simulink model "untuned_filter"  (R2021a)
settings: Solver=VariableStepAuto  StartTime=0.0  StopTime=10.0  RelTol=1e-3
libraries: xbsIndex_r4 x753
(part 1 of 2)
settings Model: Creator=s4671313  LastModifiedBy=s4671313

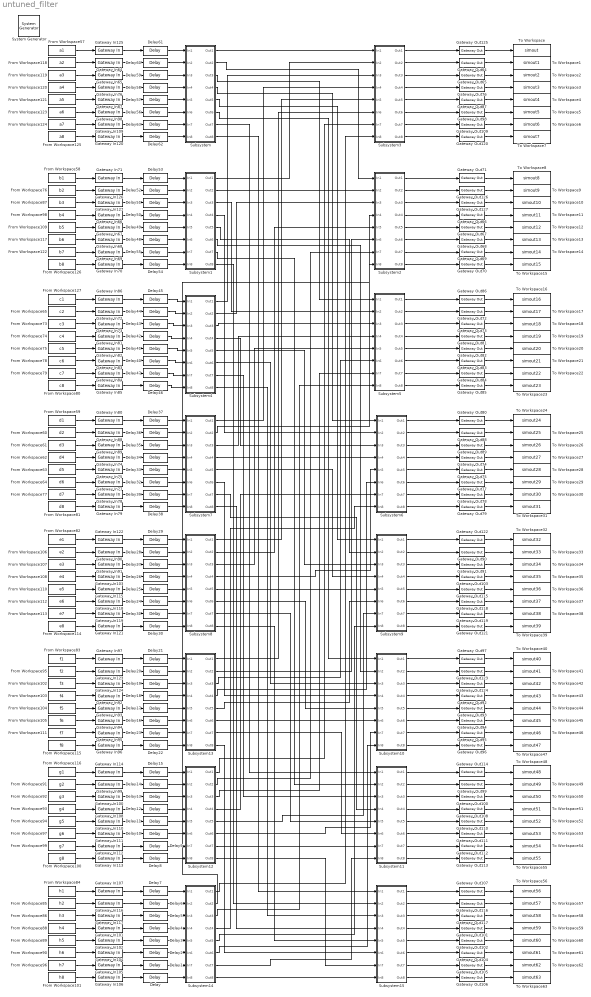
== system untuned_filter ==
  " System Generator" : xbsIndex_r4/ System Generator  Tag=genX  xilinxfamily=artix7  part=xc7a200t  speed=-2  package=fbg676  synthesis_tool=Vivado  clock_wrapper=Clock Enables  directory=./netlist  proj_type=Vivado  Synth_file=Vivado Synthesis Defaults  Impl_file=Vivado Implementation Defaults  testbench=off  simulink_period=1  sysclk_period=10  dcm_input_clock_period=10  incr_netlist=off  trim_vbits=Everywhere in SubSystem  dbl_ovrd=According to Block Masks  core_generation=According to Block Masks  run_coregen=off  deprecated_control=off  eval_field=0  block_type=sysgen
  Delay{,1..63} (64 alike) : xbsIndex_r4/Delay  rst=off  infoeditControl=Selection of Reset will increase slice count due to use of real FFs and instead of SRLs  en=off  latency=1  reg_retiming=off  dbl_ovrd=off  block_type=delay
  From Workspace100 : FromWorkspace  VariableName=g8
  From Workspace101 : FromWorkspace  VariableName=h8
  From Workspace102 : FromWorkspace  VariableName=f3
  From Workspace103 : FromWorkspace  VariableName=f4
  From Workspace104 : FromWorkspace  VariableName=f5
  From Workspace105 : FromWorkspace  VariableName=f6
  From Workspace106 : FromWorkspace  VariableName=e2
  From Workspace107 : FromWorkspace  VariableName=e3
  From Workspace108 : FromWorkspace  VariableName=e4
  From Workspace109 : FromWorkspace  VariableName=b5
  From Workspace110 : FromWorkspace  VariableName=e5
  From Workspace111 : FromWorkspace  VariableName=f7
  From Workspace112 : FromWorkspace  VariableName=e6
  From Workspace113 : FromWorkspace  VariableName=e7
  From Workspace114 : FromWorkspace  VariableName=e8
  From Workspace115 : FromWorkspace  VariableName=f8
  From Workspace116 : FromWorkspace  VariableName=g1
  From Workspace117 : FromWorkspace  VariableName=b6
  From Workspace118 : FromWorkspace  VariableName=a2
  From Workspace119 : FromWorkspace  VariableName=a3
  From Workspace120 : FromWorkspace  VariableName=a4
  From Workspace121 : FromWorkspace  VariableName=a5
  From Workspace122 : FromWorkspace  VariableName=b7
  From Workspace123 : FromWorkspace  VariableName=a6
  From Workspace124 : FromWorkspace  VariableName=a7
  From Workspace125 : FromWorkspace  VariableName=a8
  From Workspace126 : FromWorkspace  VariableName=b8
  From Workspace127 : FromWorkspace  VariableName=c1
  From Workspace57 : FromWorkspace  VariableName=a1
  From Workspace58 : FromWorkspace  VariableName=b1
  From Workspace59 : FromWorkspace  VariableName=d1
  From Workspace60 : FromWorkspace  VariableName=d2
  From Workspace61 : FromWorkspace  VariableName=d3
  From Workspace62 : FromWorkspace  VariableName=d4
  From Workspace63 : FromWorkspace  VariableName=d5
  From Workspace64 : FromWorkspace  VariableName=d6
  From Workspace65 : FromWorkspace  VariableName=c2
  From Workspace73 : FromWorkspace  VariableName=c3
  From Workspace74 : FromWorkspace  VariableName=c4
  From Workspace75 : FromWorkspace  VariableName=c5
  From Workspace76 : FromWorkspace  VariableName=b2
  From Workspace77 : FromWorkspace  VariableName=d7
  From Workspace78 : FromWorkspace  VariableName=c6
  From Workspace79 : FromWorkspace  VariableName=c7
  From Workspace80 : FromWorkspace  VariableName=c8
  From Workspace81 : FromWorkspace  VariableName=d8
  From Workspace82 : FromWorkspace  VariableName=e1
  From Workspace83 : FromWorkspace  VariableName=f1
  From Workspace84 : FromWorkspace  VariableName=h1
  From Workspace85 : FromWorkspace  VariableName=h2
  From Workspace86 : FromWorkspace  VariableName=h3
  From Workspace87 : FromWorkspace  VariableName=b3
  From Workspace88 : FromWorkspace  VariableName=h4
  From Workspace89 : FromWorkspace  VariableName=h5
  From Workspace90 : FromWorkspace  VariableName=h6
  From Workspace91 : FromWorkspace  VariableName=g2
  From Workspace92 : FromWorkspace  VariableName=g3
  From Workspace93 : FromWorkspace  VariableName=g4
  From Workspace94 : FromWorkspace  VariableName=g5
  From Workspace95 : FromWorkspace  VariableName=f2
  From Workspace96 : FromWorkspace  VariableName=h7
  From Workspace97 : FromWorkspace  VariableName=g6
  From Workspace98 : FromWorkspace  VariableName=b4
  From Workspace99 : FromWorkspace  VariableName=g7
  Gateway In{64..127} (64 alike) : xbsIndex_r4/Gateway In  gui_display_data_type=Fixed-point  arith_type="Signed  (2's comp)"  n_bits=W  bin_pt=D  preci_type=Single  exp_width=8  frac_width=24  rows=1  columns=1  quantization="Round  (unbiased: +/- Inf)"  overflow=Saturate  period=1  UseAsADC=off  ADCChannel='1'  interface=None  automatic_assignment=on  address_offset=hex2dec('00')  intf_name=''  intf_description=''  default_value=0  timing_constraint=None  locs_specified=off  LOCs={}  io_standard={}  inherit_from_input=off  hdl_port=on  dbl_ovrd=off  block_type=gatewayin
  Gateway Out{64..127} (64 alike) : xbsIndex_r4/Gateway Out  inherit_from_input=off  hdl_port=on  rows=1  columns=1  UseAsDAC=off  DACChannel='1'  interface=None  automatic_assignment=on  address_offset=hex2dec('00')  intf_name=''  intf_description=''  timing_constraint=None  locs_specified=off  LOCs={}  io_standard={}  block_type=gatewayout
  Subsystem : Subsystem
  Subsystem1 : Subsystem
  Subsystem10 : Subsystem
  Subsystem11 : Subsystem
  Subsystem12 : Subsystem
  Subsystem13 : Subsystem
  Subsystem14 : Subsystem
  Subsystem15 : Subsystem
  Subsystem2 : Subsystem
  Subsystem3 : Subsystem
  Subsystem4 : Subsystem
  Subsystem5 : Subsystem
  Subsystem6 : Subsystem
  Subsystem7 : Subsystem
  Subsystem8 : Subsystem
  Subsystem9 : Subsystem
  To Workspace : ToWorkspace  VariableName=simout  SampleTime=-1
  To Workspace1 : ToWorkspace  VariableName=simout1  SampleTime=-1
  To Workspace10 : ToWorkspace  VariableName=simout10  SampleTime=-1
  To Workspace11 : ToWorkspace  VariableName=simout11  SampleTime=-1
  To Workspace12 : ToWorkspace  VariableName=simout12  SampleTime=-1
  To Workspace13 : ToWorkspace  VariableName=simout13  SampleTime=-1
  To Workspace14 : ToWorkspace  VariableName=simout14  SampleTime=-1
  To Workspace15 : ToWorkspace  VariableName=simout15  SampleTime=-1
  To Workspace16 : ToWorkspace  VariableName=simout16  SampleTime=-1
  To Workspace17 : ToWorkspace  VariableName=simout17  SampleTime=-1
  To Workspace18 : ToWorkspace  VariableName=simout18  SampleTime=-1
  To Workspace19 : ToWorkspace  VariableName=simout19  SampleTime=-1
  To Workspace2 : ToWorkspace  VariableName=simout2  SampleTime=-1
  To Workspace20 : ToWorkspace  VariableName=simout20  SampleTime=-1
  To Workspace21 : ToWorkspace  VariableName=simout21  SampleTime=-1
  To Workspace22 : ToWorkspace  VariableName=simout22  SampleTime=-1
  To Workspace23 : ToWorkspace  VariableName=simout23  SampleTime=-1
  To Workspace24 : ToWorkspace  VariableName=simout24  SampleTime=-1
  To Workspace25 : ToWorkspace  VariableName=simout25  SampleTime=-1
  To Workspace26 : ToWorkspace  VariableName=simout26  SampleTime=-1
  To Workspace27 : ToWorkspace  VariableName=simout27  SampleTime=-1
  To Workspace28 : ToWorkspace  VariableName=simout28  SampleTime=-1
  To Workspace29 : ToWorkspace  VariableName=simout29  SampleTime=-1
  To Workspace3 : ToWorkspace  VariableName=simout3  SampleTime=-1
  To Workspace30 : ToWorkspace  VariableName=simout30  SampleTime=-1
  To Workspace31 : ToWorkspace  VariableName=simout31  SampleTime=-1
  To Workspace32 : ToWorkspace  VariableName=simout32  SampleTime=-1
  To Workspace33 : ToWorkspace  VariableName=simout33  SampleTime=-1
  To Workspace34 : ToWorkspace  VariableName=simout34  SampleTime=-1
  To Workspace35 : ToWorkspace  VariableName=simout35  SampleTime=-1
  To Workspace36 : ToWorkspace  VariableName=simout36  SampleTime=-1
  To Workspace37 : ToWorkspace  VariableName=simout37  SampleTime=-1
  To Workspace38 : ToWorkspace  VariableName=simout38  SampleTime=-1
  To Workspace39 : ToWorkspace  VariableName=simout39  SampleTime=-1
  To Workspace4 : ToWorkspace  VariableName=simout4  SampleTime=-1
  To Workspace40 : ToWorkspace  VariableName=simout40  SampleTime=-1
  To Workspace41 : ToWorkspace  VariableName=simout41  SampleTime=-1
  To Workspace42 : ToWorkspace  VariableName=simout42  SampleTime=-1
  To Workspace43 : ToWorkspace  VariableName=simout43  SampleTime=-1
  To Workspace44 : ToWorkspace  VariableName=simout44  SampleTime=-1
  To Workspace45 : ToWorkspace  VariableName=simout45  SampleTime=-1
  To Workspace46 : ToWorkspace  VariableName=simout46  SampleTime=-1
  To Workspace47 : ToWorkspace  VariableName=simout47  SampleTime=-1
  To Workspace48 : ToWorkspace  VariableName=simout48  SampleTime=-1
  To Workspace49 : ToWorkspace  VariableName=simout49  SampleTime=-1
  To Workspace5 : ToWorkspace  VariableName=simout5  SampleTime=-1
  To Workspace50 : ToWorkspace  VariableName=simout50  SampleTime=-1
  To Workspace51 : ToWorkspace  VariableName=simout51  SampleTime=-1
  To Workspace52 : ToWorkspace  VariableName=simout52  SampleTime=-1
  To Workspace53 : ToWorkspace  VariableName=simout53  SampleTime=-1
  To Workspace54 : ToWorkspace  VariableName=simout54  SampleTime=-1
  To Workspace55 : ToWorkspace  VariableName=simout55  SampleTime=-1
  To Workspace56 : ToWorkspace  VariableName=simout56  SampleTime=-1
  To Workspace57 : ToWorkspace  VariableName=simout57  SampleTime=-1
  To Workspace58 : ToWorkspace  VariableName=simout58  SampleTime=-1
  To Workspace59 : ToWorkspace  VariableName=simout59  SampleTime=-1
  To Workspace6 : ToWorkspace  VariableName=simout6  SampleTime=-1
  To Workspace60 : ToWorkspace  VariableName=simout60  SampleTime=-1
  To Workspace61 : ToWorkspace  VariableName=simout61  SampleTime=-1
  To Workspace62 : ToWorkspace  VariableName=simout62  SampleTime=-1
  To Workspace63 : ToWorkspace  VariableName=simout63  SampleTime=-1
  To Workspace7 : ToWorkspace  VariableName=simout7  SampleTime=-1
  To Workspace8 : ToWorkspace  VariableName=simout8  SampleTime=-1
  To Workspace9 : ToWorkspace  VariableName=simout9  SampleTime=-1
  wires:
  Subsystem15/5(Out5) -> Gateway Out102/1
  Subsystem15/4(Out4) -> Gateway Out101/1
  Subsystem15/3(Out3) -> Gateway Out117/1
  Subsystem15/2(Out2) -> Gateway Out116/1
  Subsystem1/8(Out8) -> Subsystem15/2(In2)
  Subsystem12/8(Out8) -> Subsystem15/7(In7)
  Subsystem8/8(Out8) -> Subsystem15/5(In5)
  Subsystem/8(Out8) -> Subsystem15/1(In1)
  Subsystem15/8(Out8) -> Gateway Out106/1
  Subsystem4/2(Out2) -> Subsystem2/3(In3)
  Delay3/1 -> Subsystem14/5(In5)
  Delay/1 -> Subsystem14/8(In8)
  Delay6/1 -> Subsystem14/2(In2)
  Subsystem14/1(Out1) -> Subsystem3/8(In8)
  Subsystem4/3(Out3) -> Subsystem5/3(In3)
  Subsystem1/7(Out7) -> Subsystem11/2(In2)
  Subsystem7/8(Out8) -> Subsystem15/4(In4)
  Subsystem13/7(Out7) -> Subsystem11/6(In6)
  Subsystem/7(Out7) -> Subsystem11/1(In1)
  Delay46/1 -> Subsystem4/8(In8)
  Subsystem4/6(Out6) -> Subsystem10/3(In3)
  Subsystem4/4(Out4) -> Subsystem6/3(In3)
  Subsystem14/3(Out3) -> Subsystem5/8(In8)
  Delay40/1 -> Subsystem4/6(In6)
  Delay43/1 -> Subsystem4/3(In3)
  Delay9/1 -> Subsystem12/7(In7)
  Delay12/1 -> Subsystem12/4(In4)
  Delay10/1 -> Subsystem12/6(In6)
  Delay14/1 -> Subsystem12/2(In2)
  Delay11/1 -> Subsystem12/5(In5)
  Subsystem12/5(Out5) -> Subsystem9/7(In7)
  Subsystem12/1(Out1) -> Subsystem3/7(In7)
  Delay41/1 -> Subsystem4/5(In5)
  Delay2/1 -> Subsystem14/6(In6)
  Subsystem14/6(Out6) -> Subsystem10/8(In8)
  Subsystem12/6(Out6) -> Subsystem10/7(In7)
  Subsystem14/4(Out4) -> Subsystem6/8(In8)
  Subsystem12/2(Out2) -> Subsystem2/7(In7)
  Subsystem8/6(Out6) -> Subsystem10/5(In5)
  Subsystem/6(Out6) -> Subsystem10/1(In1)
  Subsystem1/6(Out6) -> Subsystem10/2(In2)
  Subsystem10/8(Out8) -> Gateway Out96/1
  Subsystem10/4(Out4) -> Gateway Out92/1
  Subsystem10/2(Out2) -> Gateway Out123/1
  Subsystem10/3(Out3) -> Gateway Out124/1
  Subsystem13/6(Out6) -> Subsystem10/6(In6)
  Subsystem13/3(Out3) -> Subsystem5/6(In6)
  Subsystem13/1(Out1) -> Subsystem3/6(In6)
  Delay17/1 -> Subsystem13/5(In5)
  Delay16/1 -> Subsystem13/6(In6)
  Delay22/1 -> Subsystem13/8(In8)
  Subsystem10/1(Out1) -> Gateway Out97/1
  Delay27/1 -> Subsystem8/3(In3)
  Delay28/1 -> Subsystem8/2(In2)
  Subsystem8/1(Out1) -> Subsystem3/5(In5)
  Subsystem7/7(Out7) -> Subsystem11/4(In4)
  Delay24/1 -> Subsystem8/6(In6)
  Subsystem6/2(Out2) -> Gateway Out88/1
  Subsystem15/6(Out6) -> Gateway Out104/1
  Subsystem6/7(Out7) -> Gateway Out78/1
  Subsystem6/8(Out8) -> Gateway Out79/1
  Subsystem6/3(Out3) -> Gateway Out89/1
  Subsystem6/6(Out6) -> Gateway Out77/1
  Subsystem6/1(Out1) -> Gateway Out80/1
  Subsystem1/4(Out4) -> Subsystem6/2(In2)
  Subsystem7/4(Out4) -> Subsystem6/4(In4)
  Delay29/1 -> Subsystem8/1(In1)
  Subsystem13/5(Out5) -> Subsystem9/6(In6)
  Delay21/1 -> Subsystem13/1(In1)
  Subsystem13/4(Out4) -> Subsystem6/6(In6)
  Delay18/1 -> Subsystem13/4(In4)
  Subsystem1/1(Out1) -> Subsystem3/2(In2)
  Delay54/1 -> Subsystem1/8(In8)
  Subsystem1/2(Out2) -> Subsystem2/2(In2)
  Delay51/1 -> Subsystem1/3(In3)
  Delay55/1 -> Subsystem1/7(In7)
  Delay52/1 -> Subsystem1/2(In2)
  Subsystem5/5(Out5) -> Gateway Out82/1
  Subsystem8/4(Out4) -> Subsystem6/5(In5)
  Subsystem5/4(Out4) -> Gateway Out81/1
  Subsystem5/2(Out2) -> Gateway Out72/1
  Subsystem5/3(Out3) -> Gateway Out73/1
  Delay1/1 -> Subsystem14/7(In7)
  Delay39/1 -> Subsystem7/7(In7)
  Gateway In64/1 -> Delay60/1
  Subsystem8/2(Out2) -> Subsystem2/5(In5)
  Gateway In109/1 -> Delay63/1
  Gateway In87/1 -> Delay57/1
  Gateway In83/1 -> Delay40/1
  Gateway In85/1 -> Delay46/1
  Gateway In84/1 -> Delay47/1
  Subsystem3/3(Out3) -> Gateway Out65/1
  Gateway In72/1 -> Delay44/1
  Gateway In82/1 -> Delay41/1
  Gateway In86/1 -> Delay45/1
  Subsystem3/8(Out8) -> Gateway Out120/1
  Gateway In67/1 -> Delay49/1
  Gateway In113/1 -> Delay8/1
  Gateway In100/1 -> Delay13/1
  Gateway In114/1 -> Delay15/1
  Subsystem2/4(Out4) -> Gateway Out66/1
  Subsystem2/1(Out1) -> Gateway Out71/1
  Gateway In108/1 -> Delay12/1
  Subsystem2/8(Out8) -> Gateway Out70/1
  Gateway In112/1 -> Delay9/1
  Gateway In110/1 -> Delay11/1
  Delay44/1 -> Subsystem4/2(In2)
  Delay7/1 -> Subsystem14/1(In1)
  Gateway In99/1 -> Delay14/1
  Delay8/1 -> Subsystem12/8(In8)
  Gateway In104/1 -> Delay2/1
  Gateway In81/1 -> Delay42/1
  Gateway In102/1 -> Delay3/1
  Subsystem9/6(Out6) -> Gateway Out118/1
  Subsystem9/5(Out5) -> Gateway Out115/1
  Gateway In115/1 -> Delay25/1
  Gateway In90/1 -> Delay28/1
  Gateway In122/1 -> Delay29/1
  Gateway In116/1 -> Delay6/1
  Gateway In107/1 -> Delay7/1
  Subsystem3/6(Out6) -> Gateway Out98/1
  Gateway In88/1 -> Delay36/1
  Gateway In89/1 -> Delay35/1
  Gateway In77/1 -> Delay32/1
  Gateway In80/1 -> Delay37/1
  Gateway In78/1 -> Delay39/1
  Gateway In124/1 -> Delay19/1
  Gateway In95/1 -> Delay23/1
  Gateway In96/1 -> Delay22/1
  Gateway In127/1 -> Delay51/1
  Gateway In68/1 -> Delay48/1
  Subsystem2/5(Out5) -> Gateway Out67/1
  Subsystem/3(Out3) -> Subsystem5/1(In1)
  Subsystem/2(Out2) -> Subsystem2/1(In1)
  Subsystem6/4(Out4) -> Gateway Out74/1
  Subsystem2/6(Out6) -> Gateway Out68/1
  Delay23/1 -> Subsystem13/7(In7)
  Gateway In93/1 -> Delay17/1
  Delay63/1 -> Subsystem/7(In7)
  Delay56/1 -> Subsystem/6(In6)
  Delay57/1 -> Subsystem/5(In5)
  Subsystem13/8(Out8) -> Subsystem15/6(In6)
  Delay60/1 -> Subsystem/2(In2)
  Gateway In74/1 -> Delay34/1
  Gateway In106/1 -> Delay/1
  Subsystem7/1(Out1) -> Subsystem3/4(In4)
  Delay61/1 -> Subsystem/1(In1)
  Delay37/1 -> Subsystem7/1(In1)
  Subsystem14/8(Out8) -> Subsystem15/8(In8)
  Delay34/1 -> Subsystem7/4(In4)
  Delay31/1 -> Subsystem8/7(In7)
  Delay36/1 -> Subsystem7/2(In2)
  Subsystem5/1(Out1) -> Gateway Out86/1
  Delay62/1 -> Subsystem/8(In8)
  Subsystem3/5(Out5) -> Gateway Out87/1
  Subsystem/1(Out1) -> Subsystem3/1(In1)
  Gateway In76/1 -> Delay58/1
  Subsystem3/4(Out4) -> Gateway Out76/1
  Subsystem3/2(Out2) -> Gateway Out64/1
  Gateway In94/1 -> Delay16/1
  Subsystem15/1(Out1) -> Gateway Out107/1
  Delay45/1 -> Subsystem4/1(In1)
  Delay47/1 -> Subsystem4/7(In7)
  Gateway In125/1 -> Delay61/1
  Subsystem11/2(Out2) -> Gateway Out99/1
  Subsystem9/2(Out2) -> Gateway Out90/1
  Subsystem11/3(Out3) -> Gateway Out100/1
  Subsystem11/5(Out5) -> Gateway Out110/1
  Gateway In123/1 -> Delay20/1
  Gateway In65/1 -> Delay59/1
  Subsystem11/8(Out8) -> Gateway Out113/1
  Subsystem9/4(Out4) -> Gateway Out103/1
  Gateway In120/1 -> Delay62/1
  Subsystem11/4(Out4) -> Gateway Out108/1
  Gateway In101/1 -> Delay4/1
  Delay58/1 -> Subsystem/4(In4)
  Subsystem5/6(Out6) -> Gateway Out83/1
  Subsystem12/7(Out7) -> Subsystem11/7(In7)
  Subsystem5/8(Out8) -> Gateway Out85/1
  Delay50/1 -> Subsystem1/4(In4)
  Subsystem5/7(Out7) -> Gateway Out84/1
  Gateway In70/1 -> Delay54/1
  Delay49/1 -> Subsystem1/5(In5)
  Subsystem1/3(Out3) -> Subsystem5/2(In2)
  Delay20/1 -> Subsystem13/2(In2)
  Gateway In121/1 -> Delay30/1
  Subsystem13/2(Out2) -> Subsystem2/6(In6)
  Subsystem8/3(Out3) -> Subsystem5/5(In5)
  Subsystem14/7(Out7) -> Subsystem11/8(In8)
  Subsystem3/7(Out7) -> Gateway Out109/1
  Gateway In103/1 -> Delay26/1
  Subsystem2/3(Out3) -> Gateway Out127/1
  Subsystem9/1(Out1) -> Gateway Out122/1
  Subsystem/4(Out4) -> Subsystem6/1(In1)
  Subsystem7/5(Out5) -> Subsystem9/4(In4)
  Subsystem11/6(Out6) -> Gateway Out111/1
  Delay42/1 -> Subsystem4/4(In4)
  Gateway Out102/1 -> To Workspace60/1
  Gateway In75/1 -> Delay33/1
  Gateway Out103/1 -> To Workspace35/1
  Subsystem10/5(Out5) -> Gateway Out93/1
  From Workspace65/1 -> Gateway In72/1
  Subsystem4/7(Out7) -> Subsystem11/3(In3)
  Gateway Out104/1 -> To Workspace61/1
  Gateway In111/1 -> Delay10/1
  Gateway Out107/1 -> To Workspace56/1
  Gateway Out124/1 -> To Workspace42/1
  Gateway In98/1 -> Delay56/1
  Gateway Out64/1 -> To Workspace1/1
  Subsystem8/5(Out5) -> Subsystem9/5(In5)
  Gateway Out66/1 -> To Workspace11/1
  From Workspace121/1 -> Gateway In87/1
  From Workspace116/1 -> Gateway In114/1
  From Workspace96/1 -> Gateway In105/1
  Gateway Out96/1 -> To Workspace47/1
  From Workspace113/1 -> Gateway In119/1
  From Workspace61/1 -> Gateway In89/1
  From Workspace76/1 -> Gateway In126/1
  Gateway Out117/1 -> To Workspace58/1
  Gateway In117/1 -> Delay5/1
  Gateway Out84/1 -> To Workspace22/1
  Delay53/1 -> Subsystem1/1(In1)
  Subsystem12/3(Out3) -> Subsystem5/7(In7)
  From Workspace127/1 -> Gateway In86/1
  Gateway Out77/1 -> To Workspace29/1
  From Workspace115/1 -> Gateway In96/1
  Gateway Out116/1 -> To Workspace57/1
  From Workspace120/1 -> Gateway In76/1
  Delay15/1 -> Subsystem12/1(In1)
  From Workspace89/1 -> Gateway In102/1
  Gateway In118/1 -> Delay24/1
  Subsystem12/4(Out4) -> Subsystem6/7(In7)
  Gateway Out95/1 -> To Workspace46/1
  Gateway Out120/1 -> To Workspace7/1
  From Workspace114/1 -> Gateway In121/1
  From Workspace83/1 -> Gateway In97/1
  From Workspace62/1 -> Gateway In74/1
  Delay32/1 -> Subsystem7/6(In6)
  Gateway In79/1 -> Delay38/1
  From Workspace119/1 -> Gateway In65/1
  Gateway Out85/1 -> To Workspace23/1
  From Workspace59/1 -> Gateway In80/1
  From Workspace63/1 -> Gateway In75/1
  Gateway Out81/1 -> To Workspace19/1
  Subsystem2/7(Out7) -> Gateway Out69/1
  Subsystem15/7(Out7) -> Gateway Out105/1
  From Workspace88/1 -> Gateway In101/1
  From Workspace111/1 -> Gateway In95/1
  Gateway Out90/1 -> To Workspace33/1
  Subsystem4/1(Out1) -> Subsystem3/3(In3)
  From Workspace95/1 -> Gateway In123/1
  Subsystem4/8(Out8) -> Subsystem15/3(In3)
  From Workspace58/1 -> Gateway In71/1
  Gateway Out106/1 -> To Workspace63/1
  Subsystem8/7(Out7) -> Subsystem11/5(In5)
  From Workspace92/1 -> Gateway In100/1
  From Workspace101/1 -> Gateway In106/1
  Gateway Out99/1 -> To Workspace49/1
  Gateway Out78/1 -> To Workspace30/1
  Gateway Out83/1 -> To Workspace21/1
  From Workspace94/1 -> Gateway In110/1
  Gateway In105/1 -> Delay1/1
  From Workspace123/1 -> Gateway In98/1
  From Workspace91/1 -> Gateway In99/1
  Gateway Out93/1 -> To Workspace44/1
  From Workspace77/1 -> Gateway In78/1
  Gateway In97/1 -> Delay21/1
  From Workspace74/1 -> Gateway In81/1
  Subsystem10/7(Out7) -> Gateway Out95/1
  Gateway Out115/1 -> To Workspace36/1
  Delay26/1 -> Subsystem8/4(In4)
  Gateway Out91/1 -> To Workspace34/1
  From Workspace122/1 -> Gateway In69/1
  Gateway Out118/1 -> To Workspace37/1
  From Workspace79/1 -> Gateway In84/1
  Subsystem7/6(Out6) -> Subsystem10/4(In4)
  Gateway Out114/1 -> To Workspace48/1
  From Workspace112/1 -> Gateway In118/1
  From Workspace106/1 -> Gateway In90/1
  Gateway In119/1 -> Delay31/1
  Gateway Out108/1 -> To Workspace51/1
  Gateway Out119/1 -> To Workspace38/1
  Gateway Out105/1 -> To Workspace62/1
  Gateway Out65/1 -> To Workspace2/1
  Gateway Out101/1 -> To Workspace59/1
  Delay35/1 -> Subsystem7/3(In3)
  From Workspace107/1 -> Gateway In91/1
  From Workspace80/1 -> Gateway In85/1
  Gateway Out100/1 -> To Workspace50/1
  Gateway Out82/1 -> To Workspace20/1
  Subsystem14/5(Out5) -> Subsystem9/8(In8)
  Subsystem4/5(Out5) -> Subsystem9/3(In3)
  Gateway Out73/1 -> To Workspace18/1
  Delay5/1 -> Subsystem14/3(In3)
  From Workspace73/1 -> Gateway In73/1
  Gateway Out72/1 -> To Workspace17/1
  Gateway In73/1 -> Delay43/1
  From Workspace109/1 -> Gateway In67/1
  Subsystem6/5(Out5) -> Gateway Out75/1
  From Workspace104/1 -> Gateway In93/1
  Gateway Out92/1 -> To Workspace43/1
  From Workspace84/1 -> Gateway In107/1
  Subsystem1/5(Out5) -> Subsystem9/2(In2)
  Delay59/1 -> Subsystem/3(In3)
  Gateway Out70/1 -> To Workspace15/1
  Gateway In69/1 -> Delay55/1
  Gateway Out121/1 -> To Workspace39/1
  Subsystem/5(Out5) -> Subsystem9/1(In1)
  From Workspace105/1 -> Gateway In94/1
  From Workspace108/1 -> Gateway In103/1
  Gateway Out86/1 -> To Workspace16/1
  From Workspace110/1 -> Gateway In115/1
  Gateway Out71/1 -> To Workspace8/1
  From Workspace86/1 -> Gateway In117/1
  Subsystem9/7(Out7) -> Gateway Out119/1
  Gateway Out75/1 -> To Workspace28/1
  Gateway Out79/1 -> To Workspace31/1
  From Workspace99/1 -> Gateway In112/1
  Subsystem3/1(Out1) -> Gateway Out125/1
  Delay30/1 -> Subsystem8/8(In8)
  Gateway Out88/1 -> To Workspace25/1
  From Workspace125/1 -> Gateway In120/1
  Gateway Out122/1 -> To Workspace32/1
  Gateway In71/1 -> Delay53/1
  Subsystem7/3(Out3) -> Subsystem5/4(In4)
  Subsystem9/3(Out3) -> Gateway Out91/1
  From Workspace118/1 -> Gateway In64/1
  Gateway Out110/1 -> To Workspace52/1
  Subsystem2/2(Out2) -> Gateway Out126/1
  From Workspace100/1 -> Gateway In113/1
  Gateway Out94/1 -> To Workspace45/1
  Gateway Out67/1 -> To Workspace12/1
  Gateway Out98/1 -> To Workspace5/1
  From Workspace102/1 -> Gateway In124/1
  Gateway Out125/1 -> To Workspace/1
  Subsystem11/7(Out7) -> Gateway Out112/1
  From Workspace64/1 -> Gateway In77/1
  From Workspace87/1 -> Gateway In127/1
  Delay4/1 -> Subsystem14/4(In4)
  Gateway Out97/1 -> To Workspace40/1
  Subsystem7/2(Out2) -> Subsystem2/4(In4)
  From Workspace126/1 -> Gateway In70/1
  Subsystem10/6(Out6) -> Gateway Out94/1
  Gateway Out126/1 -> To Workspace9/1
  Subsystem11/1(Out1) -> Gateway Out114/1
  Delay33/1 -> Subsystem7/5(In5)
  From Workspace98/1 -> Gateway In66/1
  From Workspace124/1 -> Gateway In109/1
  Delay25/1 -> Subsystem8/5(In5)
  From Workspace103/1 -> Gateway In92/1
  From Workspace90/1 -> Gateway In104/1
  Subsystem14/2(Out2) -> Subsystem2/8(In8)
  Gateway Out113/1 -> To Workspace55/1
  Gateway In91/1 -> Delay27/1
  Gateway Out112/1 -> To Workspace54/1
  Gateway Out68/1 -> To Workspace13/1
  Delay13/1 -> Subsystem12/3(In3)
  Gateway Out76/1 -> To Workspace3/1
  From Workspace97/1 -> Gateway In111/1
  From Workspace93/1 -> Gateway In108/1
  From Workspace81/1 -> Gateway In79/1
  From Workspace85/1 -> Gateway In116/1
  From Workspace82/1 -> Gateway In122/1
  Gateway Out123/1 -> To Workspace41/1
  Delay38/1 -> Subsystem7/8(In8)
  Gateway Out87/1 -> To Workspace4/1
  Gateway Out111/1 -> To Workspace53/1
  Gateway In66/1 -> Delay50/1
  Subsystem9/8(Out8) -> Gateway Out121/1
  Delay48/1 -> Subsystem1/6(In6)
  Gateway Out109/1 -> To Workspace6/1
  Gateway In92/1 -> Delay18/1
  From Workspace57/1 -> Gateway In125/1
  Gateway Out74/1 -> To Workspace27/1
  Gateway Out89/1 -> To Workspace26/1
  From Workspace75/1 -> Gateway In82/1
  Gateway Out127/1 -> To Workspace10/1
  From Workspace78/1 -> Gateway In83/1
  From Workspace60/1 -> Gateway In88/1
  Delay19/1 -> Subsystem13/3(In3)
  Gateway Out80/1 -> To Workspace24/1
  Gateway Out69/1 -> To Workspace14/1
  Gateway In126/1 -> Delay52/1
  From Workspace117/1 -> Gateway In68/1

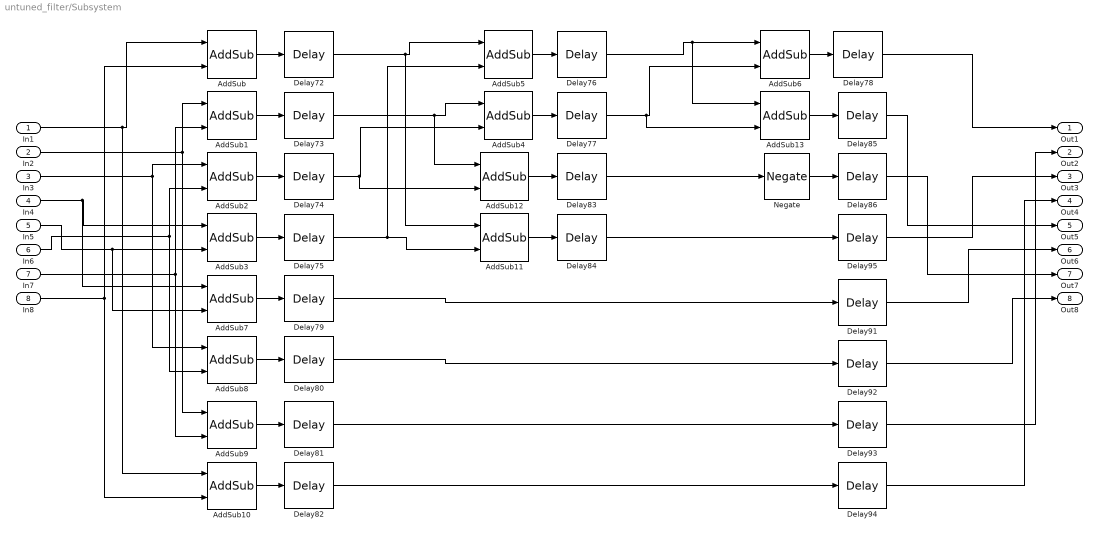
== system untuned_filter/Subsystem ==
  In1 : Inport
  In2 : Inport  Port=2
  In3 : Inport  Port=3
  In4 : Inport  Port=4
  In5 : Inport  Port=5
  In6 : Inport  Port=6
  In7 : Inport  Port=7
  In8 : Inport  Port=8
  AddSub{,1..6} (7 alike) : xbsIndex_r4/AddSub  mode=Addition  use_carryin=off  use_carryout=off  en=off  latency=0  precision=User Defined  arith_type="Signed  (2's comp)"  n_bits=Wa  bin_pt=Da  quantization="Round  (unbiased: +/- Inf)"  overflow=Saturate  use_behavioral_HDL=off  hw_selection=Fabric  pipelined=off  dbl_ovrd=off  block_type=addsub
  AddSub{7..13} (7 alike) : xbsIndex_r4/AddSub  mode=Subtraction  use_carryin=off  use_carryout=off  en=off  latency=0  precision=User Defined  arith_type="Signed  (2's comp)"  n_bits=Wa  bin_pt=Da  quantization="Round  (unbiased: +/- Inf)"  overflow=Saturate  use_behavioral_HDL=off  hw_selection=Fabric  pipelined=off  dbl_ovrd=off  block_type=addsub
  Delay{72..86,91..95} (20 alike) : xbsIndex_r4/Delay  rst=off  infoeditControl=Selection of Reset will increase slice count due to use of real FFs and instead of SRLs  en=off  latency=1  reg_retiming=off  dbl_ovrd=off  block_type=delay
  Negate : xbsIndex_r4/Negate  precision=User Defined  arith_type="Signed  (2's comp)"  n_bits=Wa  bin_pt=Da  quantization="Round  (unbiased: +/- Inf)"  overflow=Saturate  en=off  latency=0  dbl_ovrd=off  block_type=negate
  Out1 : Outport
  Out2 : Outport  Port=2
  Out3 : Outport  Port=3
  Out4 : Outport  Port=4
  Out5 : Outport  Port=5
  Out6 : Outport  Port=6
  Out7 : Outport  Port=7
  Out8 : Outport  Port=8
  wires:
  Delay86/1 -> Out7/1
  In5/1 -> AddSub7/2, AddSub3/2
  Negate/1 -> Delay86/1
  Delay74/1 -> AddSub12/2, AddSub4/2
  In8/1 -> AddSub/2, AddSub10/2
  In7/1 -> AddSub1/2, AddSub9/2
  Delay82/1 -> Delay94/1
  AddSub2/1 -> Delay74/1
  Delay84/1 -> Delay95/1
  Delay80/1 -> Delay92/1
  AddSub8/1 -> Delay80/1
  Delay76/1 -> AddSub13/1, AddSub6/1
  Delay77/1 -> AddSub13/2, AddSub6/2
  Delay92/1 -> Out8/1
  Delay72/1 -> AddSub11/1, AddSub5/1
  Delay73/1 -> AddSub12/1, AddSub4/1
  AddSub9/1 -> Delay81/1
  In6/1 -> AddSub2/2, AddSub8/2
  In4/1 -> AddSub7/1, AddSub3/1
  In3/1 -> AddSub2/1, AddSub8/1
  Delay79/1 -> Delay91/1
  In1/1 -> AddSub10/1, AddSub/1
  AddSub6/1 -> Delay78/1
  AddSub7/1 -> Delay79/1
  Delay83/1 -> Negate/1
  AddSub3/1 -> Delay75/1
  AddSub13/1 -> Delay85/1
  In2/1 -> AddSub1/1, AddSub9/1
  Delay91/1 -> Out6/1
  Delay75/1 -> AddSub5/2, AddSub11/2
  AddSub10/1 -> Delay82/1
  AddSub12/1 -> Delay83/1
  AddSub11/1 -> Delay84/1
  AddSub5/1 -> Delay76/1
  Delay78/1 -> Out1/1
  AddSub4/1 -> Delay77/1
  Delay81/1 -> Delay93/1
  AddSub1/1 -> Delay73/1
  AddSub/1 -> Delay72/1
  Delay95/1 -> Out3/1
  Delay94/1 -> Out4/1
  Delay85/1 -> Out5/1
  Delay93/1 -> Out2/1

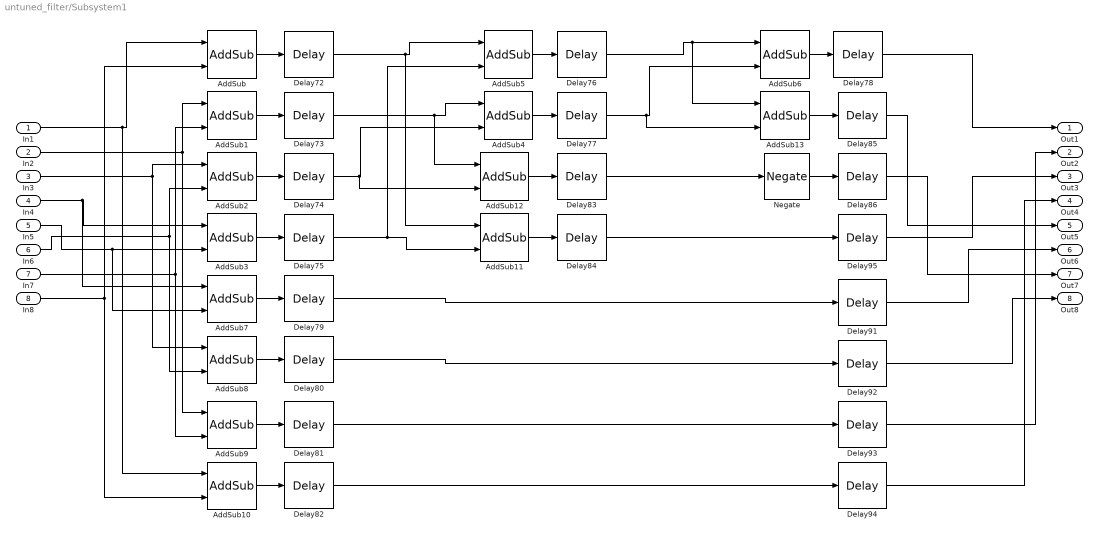
== system untuned_filter/Subsystem1 ==
  In1 : Inport
  In2 : Inport  Port=2
  In3 : Inport  Port=3
  In4 : Inport  Port=4
  In5 : Inport  Port=5
  In6 : Inport  Port=6
  In7 : Inport  Port=7
  In8 : Inport  Port=8
  AddSub{,1..6} (7 alike) : xbsIndex_r4/AddSub  mode=Addition  use_carryin=off  use_carryout=off  en=off  latency=0  precision=User Defined  arith_type="Signed  (2's comp)"  n_bits=Wa  bin_pt=Da  quantization="Round  (unbiased: +/- Inf)"  overflow=Saturate  use_behavioral_HDL=off  hw_selection=Fabric  pipelined=off  dbl_ovrd=off  block_type=addsub
  AddSub{7..13} (7 alike) : xbsIndex_r4/AddSub  mode=Subtraction  use_carryin=off  use_carryout=off  en=off  latency=0  precision=User Defined  arith_type="Signed  (2's comp)"  n_bits=Wa  bin_pt=Da  quantization="Round  (unbiased: +/- Inf)"  overflow=Saturate  use_behavioral_HDL=off  hw_selection=Fabric  pipelined=off  dbl_ovrd=off  block_type=addsub
  Delay{72..86,91..95} (20 alike) : xbsIndex_r4/Delay  rst=off  infoeditControl=Selection of Reset will increase slice count due to use of real FFs and instead of SRLs  en=off  latency=1  reg_retiming=off  dbl_ovrd=off  block_type=delay
  Negate : xbsIndex_r4/Negate  precision=User Defined  arith_type="Signed  (2's comp)"  n_bits=Wa  bin_pt=Da  quantization="Round  (unbiased: +/- Inf)"  overflow=Saturate  en=off  latency=0  dbl_ovrd=off  block_type=negate
  Out1 : Outport
  Out2 : Outport  Port=2
  Out3 : Outport  Port=3
  Out4 : Outport  Port=4
  Out5 : Outport  Port=5
  Out6 : Outport  Port=6
  Out7 : Outport  Port=7
  Out8 : Outport  Port=8
  wires:
  Delay86/1 -> Out7/1
  In5/1 -> AddSub7/2, AddSub3/2
  Negate/1 -> Delay86/1
  Delay74/1 -> AddSub12/2, AddSub4/2
  In8/1 -> AddSub/2, AddSub10/2
  In7/1 -> AddSub1/2, AddSub9/2
  Delay82/1 -> Delay94/1
  AddSub2/1 -> Delay74/1
  Delay84/1 -> Delay95/1
  Delay80/1 -> Delay92/1
  AddSub8/1 -> Delay80/1
  Delay76/1 -> AddSub13/1, AddSub6/1
  Delay77/1 -> AddSub13/2, AddSub6/2
  Delay92/1 -> Out8/1
  Delay72/1 -> AddSub11/1, AddSub5/1
  Delay73/1 -> AddSub12/1, AddSub4/1
  AddSub9/1 -> Delay81/1
  In6/1 -> AddSub2/2, AddSub8/2
  In4/1 -> AddSub7/1, AddSub3/1
  In3/1 -> AddSub2/1, AddSub8/1
  Delay79/1 -> Delay91/1
  In1/1 -> AddSub10/1, AddSub/1
  AddSub6/1 -> Delay78/1
  AddSub7/1 -> Delay79/1
  Delay83/1 -> Negate/1
  AddSub3/1 -> Delay75/1
  AddSub13/1 -> Delay85/1
  In2/1 -> AddSub1/1, AddSub9/1
  Delay91/1 -> Out6/1
  Delay75/1 -> AddSub5/2, AddSub11/2
  AddSub10/1 -> Delay82/1
  AddSub12/1 -> Delay83/1
  AddSub11/1 -> Delay84/1
  AddSub5/1 -> Delay76/1
  Delay78/1 -> Out1/1
  AddSub4/1 -> Delay77/1
  Delay81/1 -> Delay93/1
  AddSub1/1 -> Delay73/1
  AddSub/1 -> Delay72/1
  Delay95/1 -> Out3/1
  Delay94/1 -> Out4/1
  Delay85/1 -> Out5/1
  Delay93/1 -> Out2/1

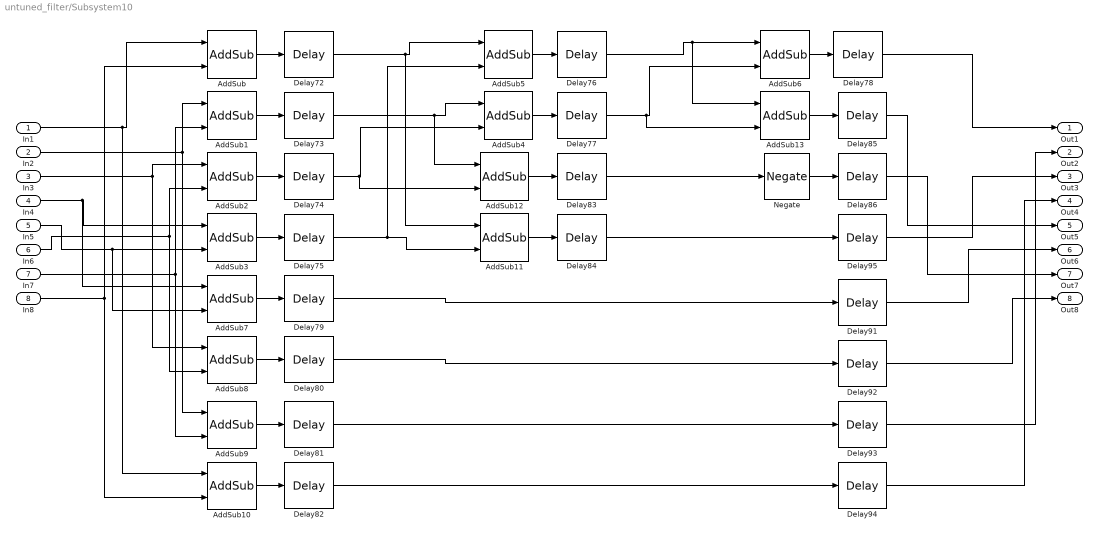
== system untuned_filter/Subsystem10 ==
  In1 : Inport
  In2 : Inport  Port=2
  In3 : Inport  Port=3
  In4 : Inport  Port=4
  In5 : Inport  Port=5
  In6 : Inport  Port=6
  In7 : Inport  Port=7
  In8 : Inport  Port=8
  AddSub{,1..6} (7 alike) : xbsIndex_r4/AddSub  mode=Addition  use_carryin=off  use_carryout=off  en=off  latency=0  precision=User Defined  arith_type="Signed  (2's comp)"  n_bits=Wa  bin_pt=Da  quantization="Round  (unbiased: +/- Inf)"  overflow=Saturate  use_behavioral_HDL=off  hw_selection=Fabric  pipelined=off  dbl_ovrd=off  block_type=addsub
  AddSub{7..13} (7 alike) : xbsIndex_r4/AddSub  mode=Subtraction  use_carryin=off  use_carryout=off  en=off  latency=0  precision=User Defined  arith_type="Signed  (2's comp)"  n_bits=Wa  bin_pt=Da  quantization="Round  (unbiased: +/- Inf)"  overflow=Saturate  use_behavioral_HDL=off  hw_selection=Fabric  pipelined=off  dbl_ovrd=off  block_type=addsub
  Delay{72..86,91..95} (20 alike) : xbsIndex_r4/Delay  rst=off  infoeditControl=Selection of Reset will increase slice count due to use of real FFs and instead of SRLs  en=off  latency=1  reg_retiming=off  dbl_ovrd=off  block_type=delay
  Negate : xbsIndex_r4/Negate  precision=User Defined  arith_type="Signed  (2's comp)"  n_bits=Wa  bin_pt=Da  quantization="Round  (unbiased: +/- Inf)"  overflow=Saturate  en=off  latency=0  dbl_ovrd=off  block_type=negate
  Out1 : Outport
  Out2 : Outport  Port=2
  Out3 : Outport  Port=3
  Out4 : Outport  Port=4
  Out5 : Outport  Port=5
  Out6 : Outport  Port=6
  Out7 : Outport  Port=7
  Out8 : Outport  Port=8
  wires:
  Delay86/1 -> Out7/1
  In5/1 -> AddSub7/2, AddSub3/2
  Negate/1 -> Delay86/1
  Delay74/1 -> AddSub12/2, AddSub4/2
  In8/1 -> AddSub/2, AddSub10/2
  In7/1 -> AddSub1/2, AddSub9/2
  Delay82/1 -> Delay94/1
  AddSub2/1 -> Delay74/1
  Delay84/1 -> Delay95/1
  Delay80/1 -> Delay92/1
  AddSub8/1 -> Delay80/1
  Delay76/1 -> AddSub13/1, AddSub6/1
  Delay77/1 -> AddSub13/2, AddSub6/2
  Delay92/1 -> Out8/1
  Delay72/1 -> AddSub11/1, AddSub5/1
  Delay73/1 -> AddSub12/1, AddSub4/1
  AddSub9/1 -> Delay81/1
  In6/1 -> AddSub2/2, AddSub8/2
  In4/1 -> AddSub7/1, AddSub3/1
  In3/1 -> AddSub2/1, AddSub8/1
  Delay79/1 -> Delay91/1
  In1/1 -> AddSub10/1, AddSub/1
  AddSub6/1 -> Delay78/1
  AddSub7/1 -> Delay79/1
  Delay83/1 -> Negate/1
  AddSub3/1 -> Delay75/1
  AddSub13/1 -> Delay85/1
  In2/1 -> AddSub1/1, AddSub9/1
  Delay91/1 -> Out6/1
  Delay75/1 -> AddSub5/2, AddSub11/2
  AddSub10/1 -> Delay82/1
  AddSub12/1 -> Delay83/1
  AddSub11/1 -> Delay84/1
  AddSub5/1 -> Delay76/1
  Delay78/1 -> Out1/1
  AddSub4/1 -> Delay77/1
  Delay81/1 -> Delay93/1
  AddSub1/1 -> Delay73/1
  AddSub/1 -> Delay72/1
  Delay95/1 -> Out3/1
  Delay94/1 -> Out4/1
  Delay85/1 -> Out5/1
  Delay93/1 -> Out2/1

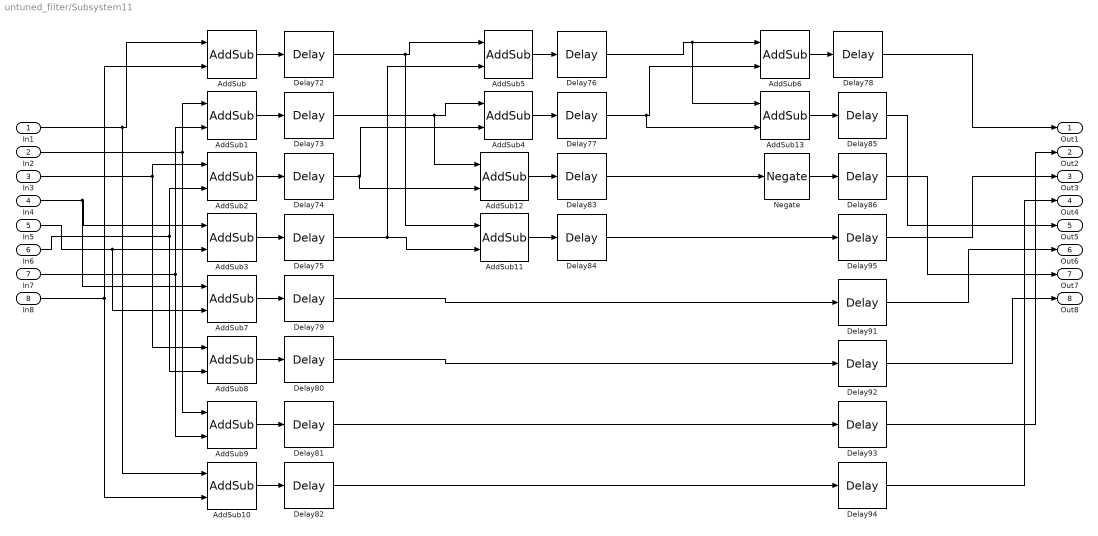
== system untuned_filter/Subsystem11 ==
  In1 : Inport
  In2 : Inport  Port=2
  In3 : Inport  Port=3
  In4 : Inport  Port=4
  In5 : Inport  Port=5
  In6 : Inport  Port=6
  In7 : Inport  Port=7
  In8 : Inport  Port=8
  AddSub{,1..6} (7 alike) : xbsIndex_r4/AddSub  mode=Addition  use_carryin=off  use_carryout=off  en=off  latency=0  precision=User Defined  arith_type="Signed  (2's comp)"  n_bits=Wa  bin_pt=Da  quantization="Round  (unbiased: +/- Inf)"  overflow=Saturate  use_behavioral_HDL=off  hw_selection=Fabric  pipelined=off  dbl_ovrd=off  block_type=addsub
  AddSub{7..13} (7 alike) : xbsIndex_r4/AddSub  mode=Subtraction  use_carryin=off  use_carryout=off  en=off  latency=0  precision=User Defined  arith_type="Signed  (2's comp)"  n_bits=Wa  bin_pt=Da  quantization="Round  (unbiased: +/- Inf)"  overflow=Saturate  use_behavioral_HDL=off  hw_selection=Fabric  pipelined=off  dbl_ovrd=off  block_type=addsub
  Delay{72..86,91..95} (20 alike) : xbsIndex_r4/Delay  rst=off  infoeditControl=Selection of Reset will increase slice count due to use of real FFs and instead of SRLs  en=off  latency=1  reg_retiming=off  dbl_ovrd=off  block_type=delay
  Negate : xbsIndex_r4/Negate  precision=User Defined  arith_type="Signed  (2's comp)"  n_bits=Wa  bin_pt=Da  quantization="Round  (unbiased: +/- Inf)"  overflow=Saturate  en=off  latency=0  dbl_ovrd=off  block_type=negate
  Out1 : Outport
  Out2 : Outport  Port=2
  Out3 : Outport  Port=3
  Out4 : Outport  Port=4
  Out5 : Outport  Port=5
  Out6 : Outport  Port=6
  Out7 : Outport  Port=7
  Out8 : Outport  Port=8
  wires:
  Delay86/1 -> Out7/1
  In5/1 -> AddSub7/2, AddSub3/2
  Negate/1 -> Delay86/1
  Delay74/1 -> AddSub12/2, AddSub4/2
  In8/1 -> AddSub/2, AddSub10/2
  In7/1 -> AddSub1/2, AddSub9/2
  Delay82/1 -> Delay94/1
  AddSub2/1 -> Delay74/1
  Delay84/1 -> Delay95/1
  Delay80/1 -> Delay92/1
  AddSub8/1 -> Delay80/1
  Delay76/1 -> AddSub13/1, AddSub6/1
  Delay77/1 -> AddSub13/2, AddSub6/2
  Delay92/1 -> Out8/1
  Delay72/1 -> AddSub11/1, AddSub5/1
  Delay73/1 -> AddSub12/1, AddSub4/1
  AddSub9/1 -> Delay81/1
  In6/1 -> AddSub2/2, AddSub8/2
  In4/1 -> AddSub7/1, AddSub3/1
  In3/1 -> AddSub2/1, AddSub8/1
  Delay79/1 -> Delay91/1
  In1/1 -> AddSub10/1, AddSub/1
  AddSub6/1 -> Delay78/1
  AddSub7/1 -> Delay79/1
  Delay83/1 -> Negate/1
  AddSub3/1 -> Delay75/1
  AddSub13/1 -> Delay85/1
  In2/1 -> AddSub1/1, AddSub9/1
  Delay91/1 -> Out6/1
  Delay75/1 -> AddSub5/2, AddSub11/2
  AddSub10/1 -> Delay82/1
  AddSub12/1 -> Delay83/1
  AddSub11/1 -> Delay84/1
  AddSub5/1 -> Delay76/1
  Delay78/1 -> Out1/1
  AddSub4/1 -> Delay77/1
  Delay81/1 -> Delay93/1
  AddSub1/1 -> Delay73/1
  AddSub/1 -> Delay72/1
  Delay95/1 -> Out3/1
  Delay94/1 -> Out4/1
  Delay85/1 -> Out5/1
  Delay93/1 -> Out2/1

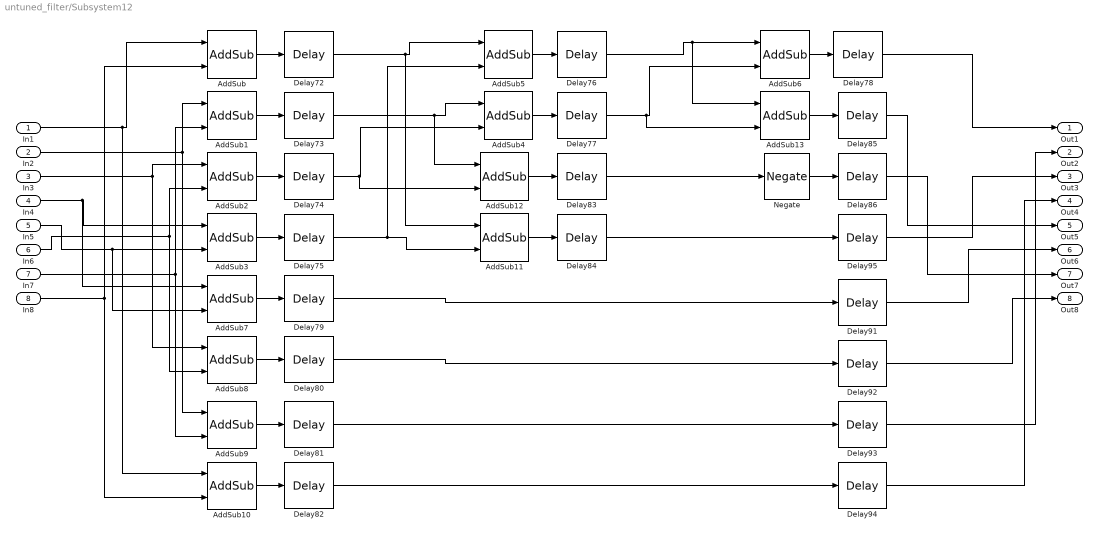
== system untuned_filter/Subsystem12 ==
  In1 : Inport
  In2 : Inport  Port=2
  In3 : Inport  Port=3
  In4 : Inport  Port=4
  In5 : Inport  Port=5
  In6 : Inport  Port=6
  In7 : Inport  Port=7
  In8 : Inport  Port=8
  AddSub{,1..6} (7 alike) : xbsIndex_r4/AddSub  mode=Addition  use_carryin=off  use_carryout=off  en=off  latency=0  precision=User Defined  arith_type="Signed  (2's comp)"  n_bits=Wa  bin_pt=Da  quantization="Round  (unbiased: +/- Inf)"  overflow=Saturate  use_behavioral_HDL=off  hw_selection=Fabric  pipelined=off  dbl_ovrd=off  block_type=addsub
  AddSub{7..13} (7 alike) : xbsIndex_r4/AddSub  mode=Subtraction  use_carryin=off  use_carryout=off  en=off  latency=0  precision=User Defined  arith_type="Signed  (2's comp)"  n_bits=Wa  bin_pt=Da  quantization="Round  (unbiased: +/- Inf)"  overflow=Saturate  use_behavioral_HDL=off  hw_selection=Fabric  pipelined=off  dbl_ovrd=off  block_type=addsub
  Delay{72..86,91..95} (20 alike) : xbsIndex_r4/Delay  rst=off  infoeditControl=Selection of Reset will increase slice count due to use of real FFs and instead of SRLs  en=off  latency=1  reg_retiming=off  dbl_ovrd=off  block_type=delay
  Negate : xbsIndex_r4/Negate  precision=User Defined  arith_type="Signed  (2's comp)"  n_bits=Wa  bin_pt=Da  quantization="Round  (unbiased: +/- Inf)"  overflow=Saturate  en=off  latency=0  dbl_ovrd=off  block_type=negate
  Out1 : Outport
  Out2 : Outport  Port=2
  Out3 : Outport  Port=3
  Out4 : Outport  Port=4
  Out5 : Outport  Port=5
  Out6 : Outport  Port=6
  Out7 : Outport  Port=7
  Out8 : Outport  Port=8
  wires:
  Delay86/1 -> Out7/1
  In5/1 -> AddSub7/2, AddSub3/2
  Negate/1 -> Delay86/1
  Delay74/1 -> AddSub12/2, AddSub4/2
  In8/1 -> AddSub/2, AddSub10/2
  In7/1 -> AddSub1/2, AddSub9/2
  Delay82/1 -> Delay94/1
  AddSub2/1 -> Delay74/1
  Delay84/1 -> Delay95/1
  Delay80/1 -> Delay92/1
  AddSub8/1 -> Delay80/1
  Delay76/1 -> AddSub13/1, AddSub6/1
  Delay77/1 -> AddSub13/2, AddSub6/2
  Delay92/1 -> Out8/1
  Delay72/1 -> AddSub11/1, AddSub5/1
  Delay73/1 -> AddSub12/1, AddSub4/1
  AddSub9/1 -> Delay81/1
  In6/1 -> AddSub2/2, AddSub8/2
  In4/1 -> AddSub7/1, AddSub3/1
  In3/1 -> AddSub2/1, AddSub8/1
  Delay79/1 -> Delay91/1
  In1/1 -> AddSub10/1, AddSub/1
  AddSub6/1 -> Delay78/1
  AddSub7/1 -> Delay79/1
  Delay83/1 -> Negate/1
  AddSub3/1 -> Delay75/1
  AddSub13/1 -> Delay85/1
  In2/1 -> AddSub1/1, AddSub9/1
  Delay91/1 -> Out6/1
  Delay75/1 -> AddSub5/2, AddSub11/2
  AddSub10/1 -> Delay82/1
  AddSub12/1 -> Delay83/1
  AddSub11/1 -> Delay84/1
  AddSub5/1 -> Delay76/1
  Delay78/1 -> Out1/1
  AddSub4/1 -> Delay77/1
  Delay81/1 -> Delay93/1
  AddSub1/1 -> Delay73/1
  AddSub/1 -> Delay72/1
  Delay95/1 -> Out3/1
  Delay94/1 -> Out4/1
  Delay85/1 -> Out5/1
  Delay93/1 -> Out2/1

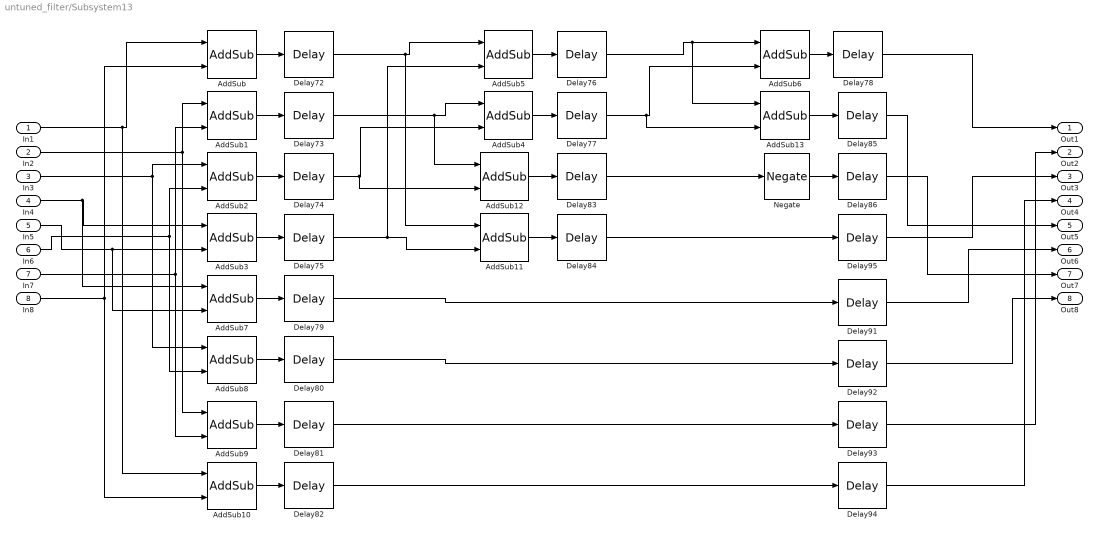
== system untuned_filter/Subsystem13 ==
  In1 : Inport
  In2 : Inport  Port=2
  In3 : Inport  Port=3
  In4 : Inport  Port=4
  In5 : Inport  Port=5
  In6 : Inport  Port=6
  In7 : Inport  Port=7
  In8 : Inport  Port=8
  AddSub{,1..6} (7 alike) : xbsIndex_r4/AddSub  mode=Addition  use_carryin=off  use_carryout=off  en=off  latency=0  precision=User Defined  arith_type="Signed  (2's comp)"  n_bits=Wa  bin_pt=Da  quantization="Round  (unbiased: +/- Inf)"  overflow=Saturate  use_behavioral_HDL=off  hw_selection=Fabric  pipelined=off  dbl_ovrd=off  block_type=addsub
  AddSub{7..13} (7 alike) : xbsIndex_r4/AddSub  mode=Subtraction  use_carryin=off  use_carryout=off  en=off  latency=0  precision=User Defined  arith_type="Signed  (2's comp)"  n_bits=Wa  bin_pt=Da  quantization="Round  (unbiased: +/- Inf)"  overflow=Saturate  use_behavioral_HDL=off  hw_selection=Fabric  pipelined=off  dbl_ovrd=off  block_type=addsub
  Delay{72..86,91..95} (20 alike) : xbsIndex_r4/Delay  rst=off  infoeditControl=Selection of Reset will increase slice count due to use of real FFs and instead of SRLs  en=off  latency=1  reg_retiming=off  dbl_ovrd=off  block_type=delay
  Negate : xbsIndex_r4/Negate  precision=User Defined  arith_type="Signed  (2's comp)"  n_bits=Wa  bin_pt=Da  quantization="Round  (unbiased: +/- Inf)"  overflow=Saturate  en=off  latency=0  dbl_ovrd=off  block_type=negate
  Out1 : Outport
  Out2 : Outport  Port=2
  Out3 : Outport  Port=3
  Out4 : Outport  Port=4
  Out5 : Outport  Port=5
  Out6 : Outport  Port=6
  Out7 : Outport  Port=7
  Out8 : Outport  Port=8
  wires:
  Delay86/1 -> Out7/1
  In5/1 -> AddSub7/2, AddSub3/2
  Negate/1 -> Delay86/1
  Delay74/1 -> AddSub12/2, AddSub4/2
  In8/1 -> AddSub/2, AddSub10/2
  In7/1 -> AddSub1/2, AddSub9/2
  Delay82/1 -> Delay94/1
  AddSub2/1 -> Delay74/1
  Delay84/1 -> Delay95/1
  Delay80/1 -> Delay92/1
  AddSub8/1 -> Delay80/1
  Delay76/1 -> AddSub13/1, AddSub6/1
  Delay77/1 -> AddSub13/2, AddSub6/2
  Delay92/1 -> Out8/1
  Delay72/1 -> AddSub11/1, AddSub5/1
  Delay73/1 -> AddSub12/1, AddSub4/1
  AddSub9/1 -> Delay81/1
  In6/1 -> AddSub2/2, AddSub8/2
  In4/1 -> AddSub7/1, AddSub3/1
  In3/1 -> AddSub2/1, AddSub8/1
  Delay79/1 -> Delay91/1
  In1/1 -> AddSub10/1, AddSub/1
  AddSub6/1 -> Delay78/1
  AddSub7/1 -> Delay79/1
  Delay83/1 -> Negate/1
  AddSub3/1 -> Delay75/1
  AddSub13/1 -> Delay85/1
  In2/1 -> AddSub1/1, AddSub9/1
  Delay91/1 -> Out6/1
  Delay75/1 -> AddSub5/2, AddSub11/2
  AddSub10/1 -> Delay82/1
  AddSub12/1 -> Delay83/1
  AddSub11/1 -> Delay84/1
  AddSub5/1 -> Delay76/1
  Delay78/1 -> Out1/1
  AddSub4/1 -> Delay77/1
  Delay81/1 -> Delay93/1
  AddSub1/1 -> Delay73/1
  AddSub/1 -> Delay72/1
  Delay95/1 -> Out3/1
  Delay94/1 -> Out4/1
  Delay85/1 -> Out5/1
  Delay93/1 -> Out2/1

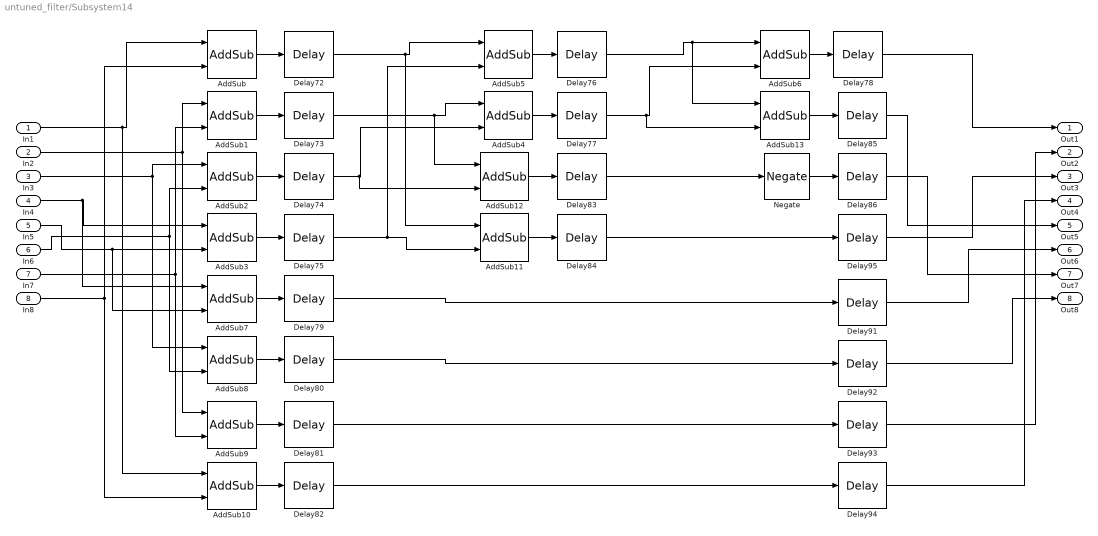
== system untuned_filter/Subsystem14 ==
  In1 : Inport
  In2 : Inport  Port=2
  In3 : Inport  Port=3
  In4 : Inport  Port=4
  In5 : Inport  Port=5
  In6 : Inport  Port=6
  In7 : Inport  Port=7
  In8 : Inport  Port=8
  AddSub{,1..6} (7 alike) : xbsIndex_r4/AddSub  mode=Addition  use_carryin=off  use_carryout=off  en=off  latency=0  precision=User Defined  arith_type="Signed  (2's comp)"  n_bits=Wa  bin_pt=Da  quantization="Round  (unbiased: +/- Inf)"  overflow=Saturate  use_behavioral_HDL=off  hw_selection=Fabric  pipelined=off  dbl_ovrd=off  block_type=addsub
  AddSub{7..13} (7 alike) : xbsIndex_r4/AddSub  mode=Subtraction  use_carryin=off  use_carryout=off  en=off  latency=0  precision=User Defined  arith_type="Signed  (2's comp)"  n_bits=Wa  bin_pt=Da  quantization="Round  (unbiased: +/- Inf)"  overflow=Saturate  use_behavioral_HDL=off  hw_selection=Fabric  pipelined=off  dbl_ovrd=off  block_type=addsub
  Delay{72..86,91..95} (20 alike) : xbsIndex_r4/Delay  rst=off  infoeditControl=Selection of Reset will increase slice count due to use of real FFs and instead of SRLs  en=off  latency=1  reg_retiming=off  dbl_ovrd=off  block_type=delay
  Negate : xbsIndex_r4/Negate  precision=User Defined  arith_type="Signed  (2's comp)"  n_bits=Wa  bin_pt=Da  quantization="Round  (unbiased: +/- Inf)"  overflow=Saturate  en=off  latency=0  dbl_ovrd=off  block_type=negate
  Out1 : Outport
  Out2 : Outport  Port=2
  Out3 : Outport  Port=3
  Out4 : Outport  Port=4
  Out5 : Outport  Port=5
  Out6 : Outport  Port=6
  Out7 : Outport  Port=7
  Out8 : Outport  Port=8
  wires:
  Delay86/1 -> Out7/1
  In5/1 -> AddSub7/2, AddSub3/2
  Negate/1 -> Delay86/1
  Delay74/1 -> AddSub12/2, AddSub4/2
  In8/1 -> AddSub/2, AddSub10/2
  In7/1 -> AddSub1/2, AddSub9/2
  Delay82/1 -> Delay94/1
  AddSub2/1 -> Delay74/1
  Delay84/1 -> Delay95/1
  Delay80/1 -> Delay92/1
  AddSub8/1 -> Delay80/1
  Delay76/1 -> AddSub13/1, AddSub6/1
  Delay77/1 -> AddSub13/2, AddSub6/2
  Delay92/1 -> Out8/1
  Delay72/1 -> AddSub11/1, AddSub5/1
  Delay73/1 -> AddSub12/1, AddSub4/1
  AddSub9/1 -> Delay81/1
  In6/1 -> AddSub2/2, AddSub8/2
  In4/1 -> AddSub7/1, AddSub3/1
  In3/1 -> AddSub2/1, AddSub8/1
  Delay79/1 -> Delay91/1
  In1/1 -> AddSub10/1, AddSub/1
  AddSub6/1 -> Delay78/1
  AddSub7/1 -> Delay79/1
  Delay83/1 -> Negate/1
  AddSub3/1 -> Delay75/1
  AddSub13/1 -> Delay85/1
  In2/1 -> AddSub1/1, AddSub9/1
  Delay91/1 -> Out6/1
  Delay75/1 -> AddSub5/2, AddSub11/2
  AddSub10/1 -> Delay82/1
  AddSub12/1 -> Delay83/1
  AddSub11/1 -> Delay84/1
  AddSub5/1 -> Delay76/1
  Delay78/1 -> Out1/1
  AddSub4/1 -> Delay77/1
  Delay81/1 -> Delay93/1
  AddSub1/1 -> Delay73/1
  AddSub/1 -> Delay72/1
  Delay95/1 -> Out3/1
  Delay94/1 -> Out4/1
  Delay85/1 -> Out5/1
  Delay93/1 -> Out2/1

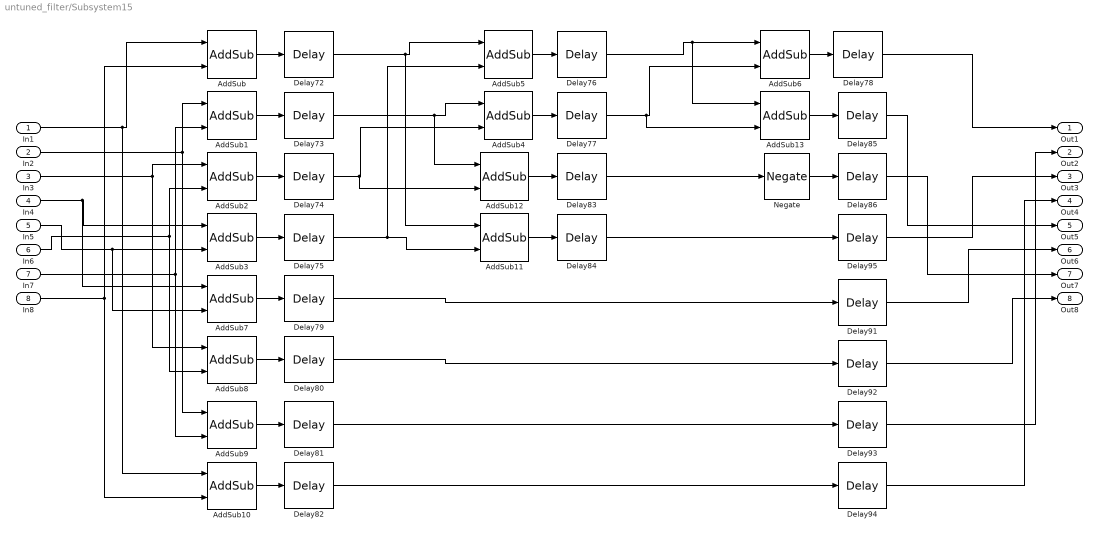
== system untuned_filter/Subsystem15 ==
  In1 : Inport
  In2 : Inport  Port=2
  In3 : Inport  Port=3
  In4 : Inport  Port=4
  In5 : Inport  Port=5
  In6 : Inport  Port=6
  In7 : Inport  Port=7
  In8 : Inport  Port=8
  AddSub{,1..6} (7 alike) : xbsIndex_r4/AddSub  mode=Addition  use_carryin=off  use_carryout=off  en=off  latency=0  precision=User Defined  arith_type="Signed  (2's comp)"  n_bits=Wa  bin_pt=Da  quantization="Round  (unbiased: +/- Inf)"  overflow=Saturate  use_behavioral_HDL=off  hw_selection=Fabric  pipelined=off  dbl_ovrd=off  block_type=addsub
  AddSub{7..13} (7 alike) : xbsIndex_r4/AddSub  mode=Subtraction  use_carryin=off  use_carryout=off  en=off  latency=0  precision=User Defined  arith_type="Signed  (2's comp)"  n_bits=Wa  bin_pt=Da  quantization="Round  (unbiased: +/- Inf)"  overflow=Saturate  use_behavioral_HDL=off  hw_selection=Fabric  pipelined=off  dbl_ovrd=off  block_type=addsub
  Delay{72..86,91..95} (20 alike) : xbsIndex_r4/Delay  rst=off  infoeditControl=Selection of Reset will increase slice count due to use of real FFs and instead of SRLs  en=off  latency=1  reg_retiming=off  dbl_ovrd=off  block_type=delay
  Negate : xbsIndex_r4/Negate  precision=User Defined  arith_type="Signed  (2's comp)"  n_bits=Wa  bin_pt=Da  quantization="Round  (unbiased: +/- Inf)"  overflow=Saturate  en=off  latency=0  dbl_ovrd=off  block_type=negate
  Out1 : Outport
  Out2 : Outport  Port=2
  Out3 : Outport  Port=3
  Out4 : Outport  Port=4
  Out5 : Outport  Port=5
  Out6 : Outport  Port=6
  Out7 : Outport  Port=7
  Out8 : Outport  Port=8
  wires:
  Delay86/1 -> Out7/1
  In5/1 -> AddSub7/2, AddSub3/2
  Negate/1 -> Delay86/1
  Delay74/1 -> AddSub12/2, AddSub4/2
  In8/1 -> AddSub/2, AddSub10/2
  In7/1 -> AddSub1/2, AddSub9/2
  Delay82/1 -> Delay94/1
  AddSub2/1 -> Delay74/1
  Delay84/1 -> Delay95/1
  Delay80/1 -> Delay92/1
  AddSub8/1 -> Delay80/1
  Delay76/1 -> AddSub13/1, AddSub6/1
  Delay77/1 -> AddSub13/2, AddSub6/2
  Delay92/1 -> Out8/1
  Delay72/1 -> AddSub11/1, AddSub5/1
  Delay73/1 -> AddSub12/1, AddSub4/1
  AddSub9/1 -> Delay81/1
  In6/1 -> AddSub2/2, AddSub8/2
  In4/1 -> AddSub7/1, AddSub3/1
  In3/1 -> AddSub2/1, AddSub8/1
  Delay79/1 -> Delay91/1
  In1/1 -> AddSub10/1, AddSub/1
  AddSub6/1 -> Delay78/1
  AddSub7/1 -> Delay79/1
  Delay83/1 -> Negate/1
  AddSub3/1 -> Delay75/1
  AddSub13/1 -> Delay85/1
  In2/1 -> AddSub1/1, AddSub9/1
  Delay91/1 -> Out6/1
  Delay75/1 -> AddSub5/2, AddSub11/2
  AddSub10/1 -> Delay82/1
  AddSub12/1 -> Delay83/1
  AddSub11/1 -> Delay84/1
  AddSub5/1 -> Delay76/1
  Delay78/1 -> Out1/1
  AddSub4/1 -> Delay77/1
  Delay81/1 -> Delay93/1
  AddSub1/1 -> Delay73/1
  AddSub/1 -> Delay72/1
  Delay95/1 -> Out3/1
  Delay94/1 -> Out4/1
  Delay85/1 -> Out5/1
  Delay93/1 -> Out2/1

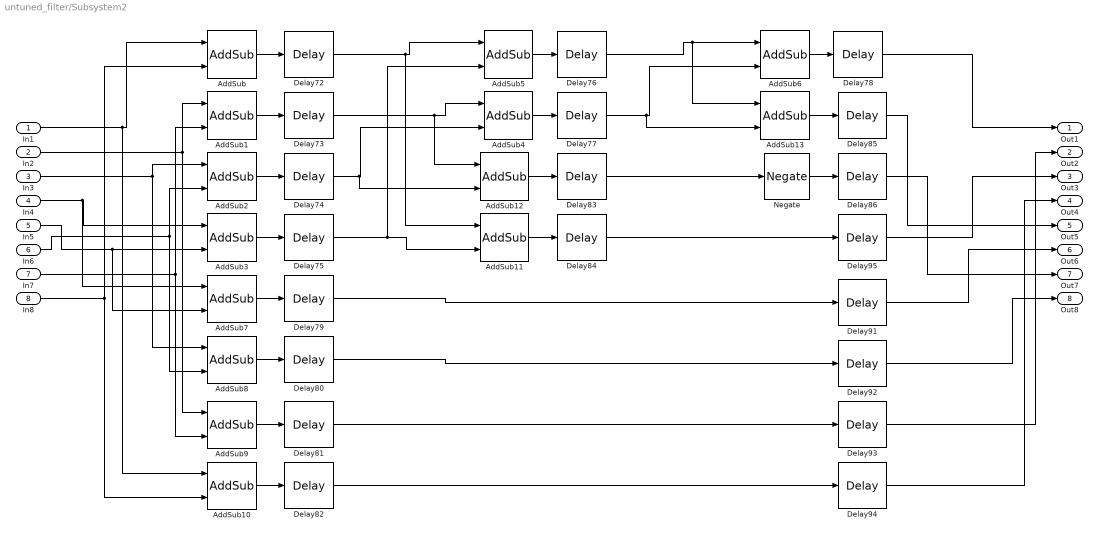
== system untuned_filter/Subsystem2 ==
  In1 : Inport
  In2 : Inport  Port=2
  In3 : Inport  Port=3
  In4 : Inport  Port=4
  In5 : Inport  Port=5
  In6 : Inport  Port=6
  In7 : Inport  Port=7
  In8 : Inport  Port=8
  AddSub{,1..6} (7 alike) : xbsIndex_r4/AddSub  mode=Addition  use_carryin=off  use_carryout=off  en=off  latency=0  precision=User Defined  arith_type="Signed  (2's comp)"  n_bits=Wa  bin_pt=Da  quantization="Round  (unbiased: +/- Inf)"  overflow=Saturate  use_behavioral_HDL=off  hw_selection=Fabric  pipelined=off  dbl_ovrd=off  block_type=addsub
  AddSub{7..13} (7 alike) : xbsIndex_r4/AddSub  mode=Subtraction  use_carryin=off  use_carryout=off  en=off  latency=0  precision=User Defined  arith_type="Signed  (2's comp)"  n_bits=Wa  bin_pt=Da  quantization="Round  (unbiased: +/- Inf)"  overflow=Saturate  use_behavioral_HDL=off  hw_selection=Fabric  pipelined=off  dbl_ovrd=off  block_type=addsub
  Delay{72..86,91..95} (20 alike) : xbsIndex_r4/Delay  rst=off  infoeditControl=Selection of Reset will increase slice count due to use of real FFs and instead of SRLs  en=off  latency=1  reg_retiming=off  dbl_ovrd=off  block_type=delay
  Negate : xbsIndex_r4/Negate  precision=User Defined  arith_type="Signed  (2's comp)"  n_bits=Wa  bin_pt=Da  quantization="Round  (unbiased: +/- Inf)"  overflow=Saturate  en=off  latency=0  dbl_ovrd=off  block_type=negate
  Out1 : Outport
  Out2 : Outport  Port=2
  Out3 : Outport  Port=3
  Out4 : Outport  Port=4
  Out5 : Outport  Port=5
  Out6 : Outport  Port=6
  Out7 : Outport  Port=7
  Out8 : Outport  Port=8
  wires:
  Delay86/1 -> Out7/1
  In5/1 -> AddSub7/2, AddSub3/2
  Negate/1 -> Delay86/1
  Delay74/1 -> AddSub12/2, AddSub4/2
  In8/1 -> AddSub/2, AddSub10/2
  In7/1 -> AddSub1/2, AddSub9/2
  Delay82/1 -> Delay94/1
  AddSub2/1 -> Delay74/1
  Delay84/1 -> Delay95/1
  Delay80/1 -> Delay92/1
  AddSub8/1 -> Delay80/1
  Delay76/1 -> AddSub13/1, AddSub6/1
  Delay77/1 -> AddSub13/2, AddSub6/2
  Delay92/1 -> Out8/1
  Delay72/1 -> AddSub11/1, AddSub5/1
  Delay73/1 -> AddSub12/1, AddSub4/1
  AddSub9/1 -> Delay81/1
  In6/1 -> AddSub2/2, AddSub8/2
  In4/1 -> AddSub7/1, AddSub3/1
  In3/1 -> AddSub2/1, AddSub8/1
  Delay79/1 -> Delay91/1
  In1/1 -> AddSub10/1, AddSub/1
  AddSub6/1 -> Delay78/1
  AddSub7/1 -> Delay79/1
  Delay83/1 -> Negate/1
  AddSub3/1 -> Delay75/1
  AddSub13/1 -> Delay85/1
  In2/1 -> AddSub1/1, AddSub9/1
  Delay91/1 -> Out6/1
  Delay75/1 -> AddSub5/2, AddSub11/2
  AddSub10/1 -> Delay82/1
  AddSub12/1 -> Delay83/1
  AddSub11/1 -> Delay84/1
  AddSub5/1 -> Delay76/1
  Delay78/1 -> Out1/1
  AddSub4/1 -> Delay77/1
  Delay81/1 -> Delay93/1
  AddSub1/1 -> Delay73/1
  AddSub/1 -> Delay72/1
  Delay95/1 -> Out3/1
  Delay94/1 -> Out4/1
  Delay85/1 -> Out5/1
  Delay93/1 -> Out2/1
